simulink model "PFC"  (R2017a)
settings: Solver=VariableStepAuto  StartTime=0.0  StopTime=0.1  MaxStep=1e-4  RelTol=1e-3
libraries: powerlib x11, powerlib_meascontrol x3
settings Model: Creator=HP  LastModifiedBy=HP

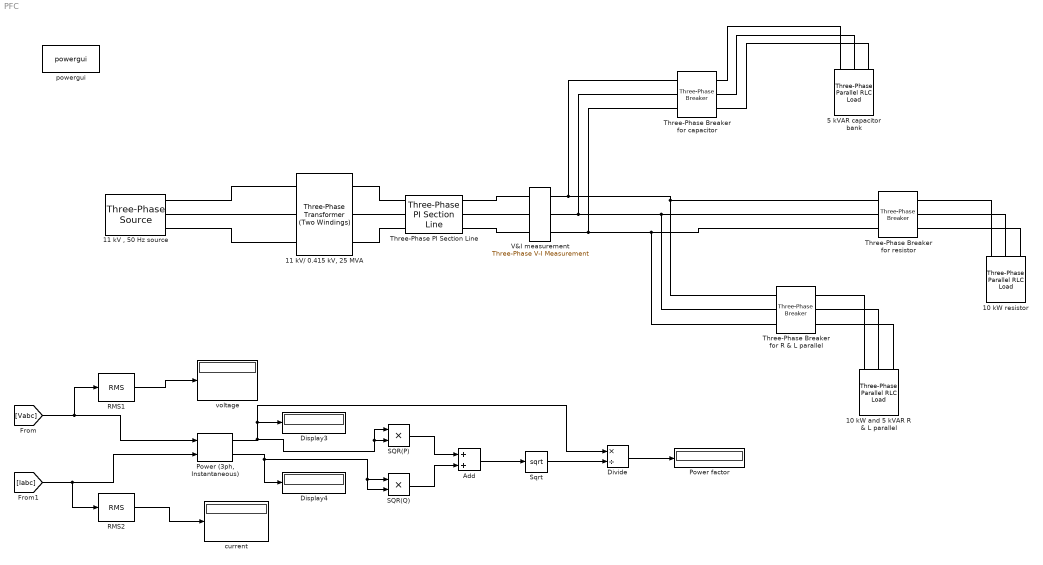
== system PFC ==
  "     5 kVAR capacitor bank" : powerlib/Elements/Three-Phase Parallel RLC Load  LConnTagsString=A|B|C  Configuration=Y (grounded)  NominalVoltage=0.415e3  Vabc=[1e3 1e3 1e3]  Vabcp=[1e3 1e3 1e3]  NominalFrequency=50  UnbalancedPower=off  ActivePower=0  InductivePower=0  CapacitivePower=5e3  Pabc=[10e3 9e3 11e3]  QLabc=[100 90 110]  QCabc=[100 90 110]  Pabcp=[10e3 9e3 11e3]  QLabcp=[100 90 110]  QCabcp=[100 90 110]  Measurements=None  LoadType=constant Z
  "    10 kW resistor" : powerlib/Elements/Three-Phase Parallel RLC Load  LConnTagsString=A|B|C  Configuration=Y (grounded)  NominalVoltage=0.415e3  Vabc=[1e3 1e3 1e3]  Vabcp=[1e3 1e3 1e3]  NominalFrequency=50  UnbalancedPower=off  ActivePower=10e3  InductivePower=0  CapacitivePower=0  Pabc=[10e3 9e3 11e3]  QLabc=[100 90 110]  QCabc=[100 90 110]  Pabcp=[10e3 9e3 11e3]  QLabcp=[100 90 110]  QCabcp=[100 90 110]  Measurements=None  LoadType=constant Z
  "   10 kW and 5 kVAR R & L parallel " : powerlib/Elements/Three-Phase Parallel RLC Load  LConnTagsString=A|B|C  Configuration=Y (grounded)  NominalVoltage=0.415e3  Vabc=[1e3 1e3 1e3]  Vabcp=[1e3 1e3 1e3]  NominalFrequency=50  UnbalancedPower=off  ActivePower=10e3  InductivePower=5e3  CapacitivePower=0  Pabc=[10e3 9e3 11e3]  QLabc=[100 90 110]  QCabc=[100 90 110]  Pabcp=[10e3 9e3 11e3]  QLabcp=[100 90 110]  QCabcp=[100 90 110]  Measurements=None  LoadType=constant Z
  "11 kV , 50 Hz source" : powerlib/Electrical Sources/Three-Phase Source  InternalConnection=Yg  VoltagePhases=off  Voltage=11e3  PhaseAngle=0  Voltage_phases=[25e3 25e3 25e3]/sqrt(3)  PhaseAngles_phases=[0 -120 +120]  Frequency=50  NonIdealSource=on  SpecifyImpedance=off  Resistance=0.8929  Inductance=16.58e-3  ShortCircuitLevel=100e6  BaseVoltage=25e3  XRratio=7  BusType=swing  Pref=10e3  Qref=0  Prefabc=[10e3, 10e3, 10e3]  Qrefabc=[0, 0, 0]  Qmin=-inf  Qmax=inf
  "11 kV/ 0.415 kV, 25 MVA" : powerlib/Elements/Three-Phase Transformer (Two Windings)  Winding1Connection=Yg  Winding2Connection=Yg  CoreType=Three single-phase transformers  SetSaturation=off  Hysteresis=off  DataFile='hysteresis'  SetInitialFlux=off  Measurements=None  UNITS=pu  NominalPower=[ 25e6 , 50 ]  Winding1=[ 11e3 , 0.002 , 0.08 ]  Winding2=[ 0.415e3 , 0.002 , 0.08 ]  Rm=500  Lm=500  L0=0.5  Saturation=[ 0,0 ; 0.0024,1.2 ; 1.0,1.52 ]  InitialFluxes=[ 0.8 , -0.8 , 0.7 ]  MoreParameters=off  BreakLoop=off  DataType=off  TransfoNumber=1
  Add : Sum
  Display3 : Display
  Display4 : Display
  Divide : Product  Inputs=*/
  "Power (3ph, Instantaneous)" : powerlib_meascontrol/Measurements/Power (3ph, Instantaneous)
      settings: SourceProductName=Simscape Power Systems
  Power factor : Display
      settings: Decimation=3
  RMS1 : powerlib_meascontrol/Measurements/RMS  TrueRMS=on  Freq=60  RMSInit=120  Ts=0
  RMS2 : powerlib_meascontrol/Measurements/RMS  TrueRMS=on  Freq=60  RMSInit=120  Ts=0
  SQR(P) : Product
  SQR(Q) : Product
  Sqrt : Sqrt  SaturateOnIntegerOverflow=on
  Three-Phase PI Section Line : powerlib/Elements/Three-Phase PI Section Line  LConnTagsString=a|b|c  RConnTagsString=A|B|C  Frequency=50  Resistances=[ 0.01273 0.3864]  Inductances="[ 0.9337e-3  4.1264e-3]"  Capacitances=[12.74e-9 7.751e-9]  Length=0.01
      settings: SourceProductName=Simscape Power Systems
  Three-Phase Breaker for R & L parallel : powerlib/Elements/Three-Phase Breaker  InitialState=closed  SwitchA=on  SwitchB=on  SwitchC=on  SwitchTimes="[1/60  5/60]"  External=off  BreakerResistance=0.01  SnubberResistance=1e6  SnubberCapacitance=inf  Measurements=None
  Three-Phase Breaker for capacitor : powerlib/Elements/Three-Phase Breaker  InitialState=closed  SwitchA=on  SwitchB=on  SwitchC=on  SwitchTimes="[1/60  5/60]"  External=off  BreakerResistance=0.01  SnubberResistance=1e6  SnubberCapacitance=inf  Measurements=None
  Three-Phase Breaker for resistor : powerlib/Elements/Three-Phase Breaker  InitialState=open  SwitchA=on  SwitchB=on  SwitchC=on  SwitchTimes="[1/60  5/60]"  External=off  BreakerResistance=0.01  SnubberResistance=1e6  SnubberCapacitance=inf  Measurements=None
  V&I measurement : powerlib/Measurements/Three-Phase V-I Measurement  VoltageMeasurement=phase-to-ground  SetLabelV=on  LabelV=Vabc  Vpu=off  VpuLL=off  CurrentMeasurement=yes  SetLabelI=on  LabelI=Iabc  Ipu=off  Pbase=100e6  Vbase=500e3  OutputType=Complex  PhasorSimulation=off  PSBequivalent=0
  current : Display
  powergui : powerlib/powergui  Priority=1  SimulationMode=Continuous  SampleTime=50e-6  frequency=60  Iterations=50  frequencyindice=50  Pbase=100e6  ErrMax=1e-4  UnitsV=kV  UnitsW=MW  buscounter=0  FunctionMessages=off  echomessages=off  EnableUseOfTLC=off  CurrentSourceSwitches=off  DisableSnubberDevices=off  DisableRonSwitches=off  DisableVfSwitches=off  DisplayEquations=off  SolverType=Tustin/Backward Euler (TBE)  Interpol=off  ExternalGateDelay=off  methode=off  Ts=100  x0status=blocks  SPID=on  SwTol=0  HookPort=off  RestoreLinks=warning  ResistiveCurrentMeasurement=off  Frange=[0:2:500]  Ylog=off  Xlog=on  ShowGrid=off  save=off  variable=ZData  structure=0  ZoomFFT=off  StartTime=0.0  cycles=1  DisplayStyle=1  fundamental=60  FreqAxis=off  MaxFrequency=1000  frequencyindicesteady=1  RmsSteady=1  display=off
  voltage : Display
  wires:
  [Vabc] -> RMS1/1, "Power (3ph, Instantaneous)"/1
  [Iabc] -> RMS2/1, "Power (3ph, Instantaneous)"/2
  RMS1/1 -> voltage/1
  RMS2/1 -> current/1
  "Power (3ph, Instantaneous)"/1 -> SQR(P)/2, SQR(P)/1, Divide/1, Display3/1
  "Power (3ph, Instantaneous)"/2 -> SQR(Q)/2, SQR(Q)/1, Display4/1
  SQR(P)/1 -> Add/1
  SQR(Q)/1 -> Add/2
  Add/1 -> Sqrt/1
  Sqrt/1 -> Divide/2
  Divide/1 -> Power factor/1
  connections:
  "11 kV , 50 Hz source"/RConn1 -- "11 kV/ 0.415 kV, 25 MVA"/LConn1
  "11 kV , 50 Hz source"/RConn2 -- "11 kV/ 0.415 kV, 25 MVA"/LConn2
  "11 kV , 50 Hz source"/RConn3 -- "11 kV/ 0.415 kV, 25 MVA"/LConn3
  Three-Phase PI Section Line/LConn2 -- "11 kV/ 0.415 kV, 25 MVA"/RConn2
  "11 kV/ 0.415 kV, 25 MVA"/RConn1 -- Three-Phase PI Section Line/LConn1
  "11 kV/ 0.415 kV, 25 MVA"/RConn3 -- Three-Phase PI Section Line/LConn3
  V&I measurement/LConn2 -- Three-Phase PI Section Line/RConn2
  Three-Phase PI Section Line/RConn1 -- V&I measurement/LConn1
  Three-Phase PI Section Line/RConn3 -- V&I measurement/LConn3
  V&I measurement/RConn1 -- Three-Phase Breaker for R & L parallel/LConn1 -- Three-Phase Breaker for resistor/LConn1 -- Three-Phase Breaker for capacitor/LConn1
  V&I measurement/RConn2 -- Three-Phase Breaker for R & L parallel/LConn2 -- Three-Phase Breaker for resistor/LConn2 -- Three-Phase Breaker for capacitor/LConn2
  V&I measurement/RConn3 -- Three-Phase Breaker for R & L parallel/LConn3 -- Three-Phase Breaker for resistor/LConn3 -- Three-Phase Breaker for capacitor/LConn3
  Three-Phase Breaker for capacitor/RConn1 -- "     5 kVAR capacitor bank"/LConn1
  Three-Phase Breaker for capacitor/RConn2 -- "     5 kVAR capacitor bank"/LConn2
  Three-Phase Breaker for capacitor/RConn3 -- "     5 kVAR capacitor bank"/LConn3
  Three-Phase Breaker for resistor/RConn1 -- "    10 kW resistor"/LConn1
  Three-Phase Breaker for resistor/RConn3 -- "    10 kW resistor"/LConn3
  Three-Phase Breaker for resistor/RConn2 -- "    10 kW resistor"/LConn2
  Three-Phase Breaker for R & L parallel/RConn2 -- "   10 kW and 5 kVAR R & L parallel "/LConn2
  Three-Phase Breaker for R & L parallel/RConn3 -- "   10 kW and 5 kVAR R & L parallel "/LConn3
  Three-Phase Breaker for R & L parallel/RConn1 -- "   10 kW and 5 kVAR R & L parallel "/LConn1
